simulink model "Sim_DDPG"  (R2025a)
settings: Solver=ode1  StartTime=0.0  StopTime=Tf  FixedStep=Ts_Sim  RelTol=1e-3
undefined symbols (not defined in the file): p_IC, phi_IC, phi_limit, pqr_Limit, psi_IC, psi_limit, q_IC, r_IC, theta_IC, theta_limit, Ts_Sim, u_IC, uvw_Limit, v_IC, w_IC, x_IC, xy_Limit, y_IC, z_IC, z_Limit
libraries: rllib x2
settings Model: Creator=nt488543  LastModifiedBy=nt488543

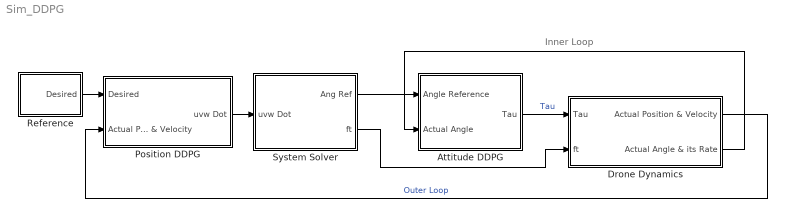
== system Sim_DDPG ==
  note: Inner Loop
  Attitude DDPG : Subsystem
  Drone Dynamics : Subsystem
  Position DDPG : Subsystem
  Reference : Subsystem
  System Solver : Subsystem
  wires:
  Reference/1(Desired) -> Position DDPG/1(Desired)
  Attitude DDPG/1(Tau) -> Drone Dynamics/1(Tau)  "Tau"
  Drone Dynamics/1(Actual Position & Velocity) -> Position DDPG/2(Actual Position & Velocity)  "Outer Loop"
  Drone Dynamics/2(Actual Angle & its Rate) -> Attitude DDPG/2(Actual Angle)
  Position DDPG/1(uvw Dot) -> System Solver/1(uvw Dot)
  System Solver/1(Ang Ref) -> Attitude DDPG/1(Angle Reference)
  System Solver/2(ft) -> Drone Dynamics/2(ft)

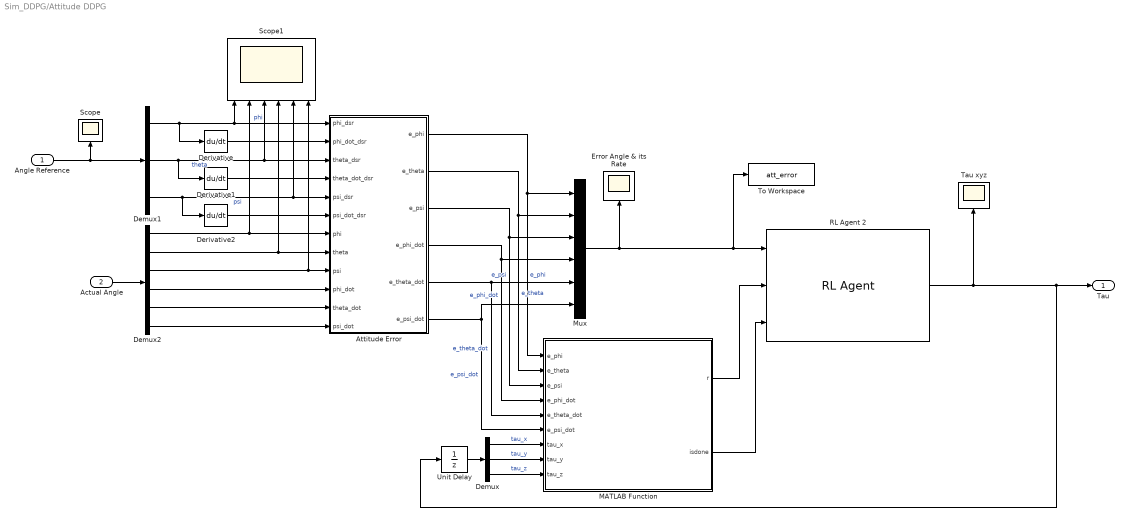
== system Sim_DDPG/Attitude DDPG ==
  Angle Reference : Inport
  Actual Angle : Inport  Port=2
  Attitude Error : MATLAB Function  TreatAsAtomicUnit=on
  Demux : Demux  Outputs=3
  Demux1 : Demux  Outputs=3
  Demux2 : Demux  Outputs=6
  Derivative : Derivative
  Derivative1 : Derivative
  Derivative2 : Derivative
  Error Angle & its Rate : Scope
      settings: ActiveDisplayYMinimum=-3.5181599273654109  ActiveDisplayYMaximum=2.1435969273697308  DataLoggingVariableName=ScopeData12
  MATLAB Function : MATLAB Function  TreatAsAtomicUnit=on
  Mux : Mux  Inputs=6
  RL Agent 2 : rllib/RL Agent  Agent=agent2  ExternalActionAsInput=off  ProvideLastAction=off  ProvideCumRwd=off  TreatAsDirectFeedthrough=on  UseStrictObservationDataTypes=off
  Scope : Scope
      settings: ActiveDisplayYMinimum=-0.07573  ActiveDisplayYMaximum=0.06612  DataLoggingVariableName=ScopeData5
  Scope1 : Scope  NumInputPorts=6
      settings: ActiveDisplayYMinimum=-0.31729729958403707  ActiveDisplayYMaximum=0.34620944603052173  DataLoggingVariableName=ScopeData6
  Tau xyz : Scope
      settings: ActiveDisplayYMinimum=-2.4987406879663467  ActiveDisplayYMaximum=2.4991613775491714  DataLoggingVariableName=ScopeData11
  To Workspace : ToWorkspace  VariableName=att_error  SampleTime=Ts_Sim
  Unit Delay : UnitDelay  SampleTime=Ts_Sim  HasFrameUpgradeWarning=on
  Tau : Outport
  wires:
  MATLAB Function/1(r) -> RL Agent 2/2
  Mux/1 -> To Workspace/1, RL Agent 2/1, Error Angle & its Rate/1
  Attitude Error/1(e_phi) -> Mux/1, MATLAB Function/1(e_phi)  "e_phi"
  Attitude Error/2(e_theta) -> Mux/2, MATLAB Function/2(e_theta)  "e_theta"
  Attitude Error/3(e_psi) -> Mux/3, MATLAB Function/3(e_psi)  "e_psi"
  Attitude Error/4(e_phi_dot) -> Mux/4, MATLAB Function/4(e_phi_dot)  "e_phi_dot"
  Attitude Error/5(e_theta_dot) -> MATLAB Function/5(e_theta_dot), Mux/5  "e_theta_dot"
  Attitude Error/6(e_psi_dot) -> MATLAB Function/6(e_psi_dot), Mux/6  "e_psi_dot"
  MATLAB Function/2(isdone) -> RL Agent 2/3
  Demux/1 -> MATLAB Function/7(tau_x)  "tau_x"
  Demux/2 -> MATLAB Function/8(tau_y)  "tau_y"
  Demux/3 -> MATLAB Function/9(tau_z)  "tau_z"
  RL Agent 2/1 -> Unit Delay/1, Tau/1, Tau xyz/1
  Demux2/1 -> Scope1/2, Attitude Error/7(phi)
  Demux2/2 -> Scope1/4, Attitude Error/8(theta)
  Demux2/3 -> Attitude Error/9(psi), Scope1/6
  Demux2/4 -> Attitude Error/10(phi_dot)
  Demux2/5 -> Attitude Error/11(theta_dot)
  Demux2/6 -> Attitude Error/12(psi_dot)
  Actual Angle/1 -> Demux2/1
  Unit Delay/1 -> Demux/1
  Demux1/1 -> Derivative/1, Attitude Error/1(phi_dsr), Scope1/1  "phi"
  Demux1/3 -> Derivative2/1, Attitude Error/5(psi_dsr), Scope1/5  "psi"
  Demux1/2 -> Derivative1/1, Attitude Error/3(theta_dsr), Scope1/3  "theta"
  Angle Reference/1 -> Demux1/1, Scope/1
  Derivative/1 -> Attitude Error/2(phi_dot_dsr)
  Derivative1/1 -> Attitude Error/4(theta_dot_dsr)
  Derivative2/1 -> Attitude Error/6(psi_dot_dsr)

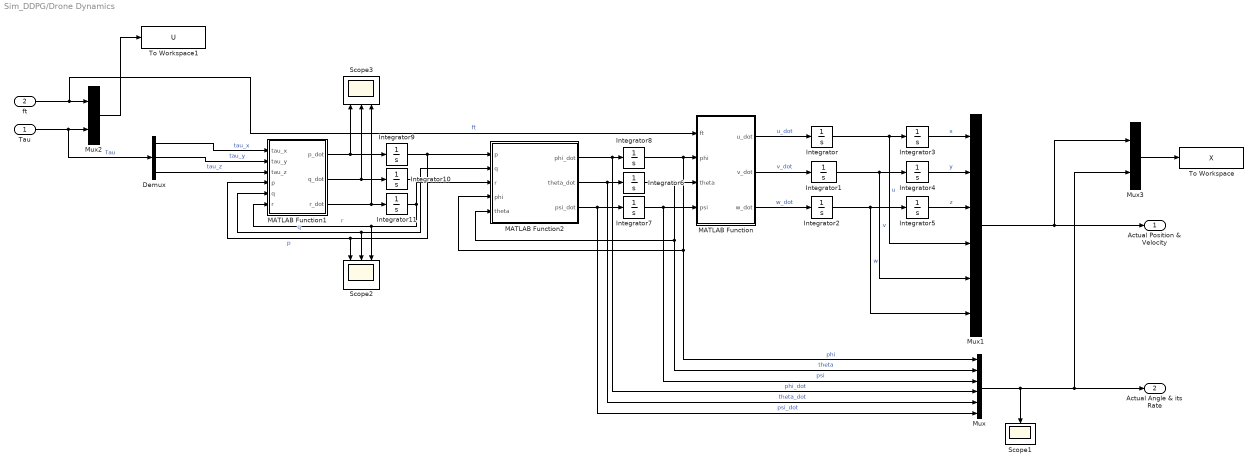
== system Sim_DDPG/Drone Dynamics ==
  Tau : Inport
  ft : Inport  Port=2
  Demux : Demux  Outputs=3
  Integrator : Integrator  InitialCondition=u_IC  UpperSaturationLimit=uvw_Limit  LowerSaturationLimit=-uvw_Limit
  Integrator1 : Integrator  InitialCondition=v_IC  UpperSaturationLimit=uvw_Limit  LowerSaturationLimit=-uvw_Limit
  Integrator10 : Integrator  InitialCondition=q_IC  UpperSaturationLimit=pqr_Limit  LowerSaturationLimit=-pqr_Limit
  Integrator11 : Integrator  InitialCondition=r_IC  UpperSaturationLimit=pqr_Limit  LowerSaturationLimit=-pqr_Limit
  Integrator2 : Integrator  InitialCondition=w_IC  UpperSaturationLimit=uvw_Limit  LowerSaturationLimit=-uvw_Limit
  Integrator3 : Integrator  InitialCondition=x_IC  UpperSaturationLimit=xy_Limit  LowerSaturationLimit=-xy_Limit
  Integrator4 : Integrator  InitialCondition=y_IC  UpperSaturationLimit=xy_Limit  LowerSaturationLimit=-xy_Limit
  Integrator5 : Integrator  InitialCondition=z_IC  UpperSaturationLimit=z_Limit  LowerSaturationLimit=-z_Limit
  Integrator6 : Integrator  InitialCondition=theta_IC  UpperSaturationLimit=theta_limit  LowerSaturationLimit=-theta_limit  WrappedStateUpperValue=pi/2  WrappedStateLowerValue=-pi/2
  Integrator7 : Integrator  InitialCondition=psi_IC  UpperSaturationLimit=psi_limit  LowerSaturationLimit=-psi_limit
  Integrator8 : Integrator  InitialCondition=phi_IC  UpperSaturationLimit=phi_limit  LowerSaturationLimit=-phi_limit
  Integrator9 : Integrator  InitialCondition=p_IC  UpperSaturationLimit=pqr_Limit  LowerSaturationLimit=-pqr_Limit
  MATLAB Function : MATLAB Function  TreatAsAtomicUnit=on
  MATLAB Function1 : MATLAB Function  TreatAsAtomicUnit=on
  MATLAB Function2 : MATLAB Function  TreatAsAtomicUnit=on
  Mux : Mux  Inputs=6
  Mux1 : Mux  Inputs=6
  Mux2 : Mux  Inputs=2
  Mux3 : Mux  Inputs=2
  Scope1 : Scope
      settings: ActiveDisplayYMinimum=-0.79782557910284335  ActiveDisplayYMaximum=0.70695961840012789  DataLoggingVariableName=ScopeData2
  Scope2 : Scope  NumInputPorts=3
      settings: ActiveDisplayYMinimum=-0.95183  ActiveDisplayYMaximum=0.89979  DataLoggingVariableName=ScopeData3
  Scope3 : Scope  NumInputPorts=3
      settings: ActiveDisplayYMinimum=-1  ActiveDisplayYMaximum=1  DataLoggingVariableName=ScopeData4
  To Workspace : ToWorkspace  VariableName=X  SampleTime=Ts_Sim
  To Workspace1 : ToWorkspace  VariableName=U  SampleTime=Ts_Sim
  Actual Position & Velocity : Outport
  Actual Angle & its Rate : Outport  Port=2
  wires:
  Integrator4/1 -> Mux1/2  "y"
  MATLAB Function1/3(r_dot) -> Scope3/3, Integrator11/1
  MATLAB Function1/1(p_dot) -> Scope3/1, Integrator9/1
  Integrator3/1 -> Mux1/1  "x"
  Integrator5/1 -> Mux1/3  "z"
  Integrator1/1 -> Mux1/5, Integrator4/1  "v"
  Demux/2 -> MATLAB Function1/2(tau_y)  "tau_y"
  Integrator9/1 -> MATLAB Function1/4(p), Scope2/1, MATLAB Function2/1(p)  "p"
  Integrator11/1 -> MATLAB Function1/6(r), Scope2/3, MATLAB Function2/3(r)  "r"
  Integrator2/1 -> Mux1/6, Integrator5/1  "w"
  Integrator/1 -> Mux1/4, Integrator3/1  "u"
  Integrator7/1 -> Mux/3, MATLAB Function/4(psi)  "psi"
  Integrator8/1 -> Mux/1, MATLAB Function2/4(phi), MATLAB Function/2(phi)  "phi"
  Integrator6/1 -> MATLAB Function/3(theta), Mux/2, MATLAB Function2/5(theta)  "theta"
  Integrator10/1 -> MATLAB Function2/2(q), MATLAB Function1/5(q), Scope2/2  "q"
  Demux/3 -> MATLAB Function1/3(tau_z)  "tau_z"
  MATLAB Function/3(w_dot) -> Integrator2/1  "w_dot"
  MATLAB Function/1(u_dot) -> Integrator/1  "u_dot"
  MATLAB Function/2(v_dot) -> Integrator1/1  "v_dot"
  MATLAB Function1/2(q_dot) -> Scope3/2, Integrator10/1
  Demux/1 -> MATLAB Function1/1(tau_x)  "tau_x"
  MATLAB Function2/1(phi_dot) -> Mux/4, Integrator8/1  "phi_dot"
  MATLAB Function2/2(theta_dot) -> Mux/5, Integrator6/1  "theta_dot"
  MATLAB Function2/3(psi_dot) -> Mux/6, Integrator7/1  "psi_dot"
  Mux/1 -> Mux3/2, Actual Angle & its Rate/1, Scope1/1
  Mux1/1 -> Mux3/1, Actual Position & Velocity/1
  Mux2/1 -> To Workspace1/1
  ft/1 -> MATLAB Function/1(ft), Mux2/1  "ft"
  Tau/1 -> Demux/1, Mux2/2  "Tau"
  Mux3/1 -> To Workspace/1

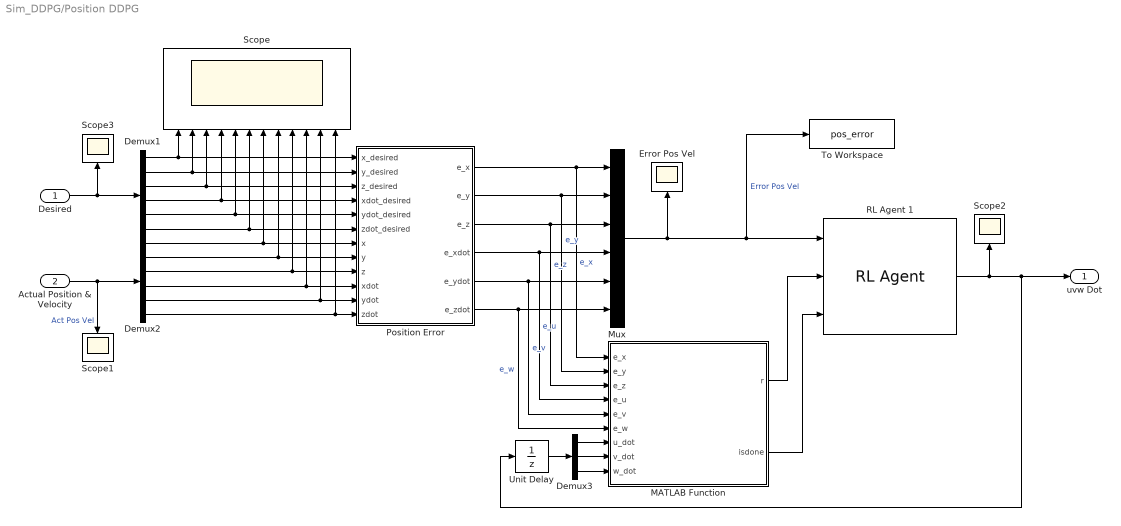
== system Sim_DDPG/Position DDPG ==
  Desired : Inport
  Actual Position & Velocity : Inport  Port=2
  Demux1 : Demux  Outputs=6
  Demux2 : Demux  Outputs=6
  Demux3 : Demux  Outputs=3
  Error Pos Vel : Scope
      settings: ActiveDisplayYMinimum=-1.3710264936743408  ActiveDisplayYMaximum=0.56946492466600562  DataLoggingVariableName=Error
  MATLAB Function : MATLAB Function  TreatAsAtomicUnit=on
  Mux : Mux  Inputs=6
  Position Error : MATLAB Function  TreatAsAtomicUnit=on
  RL Agent 1 : rllib/RL Agent  Agent=agent  ExternalActionAsInput=off  ProvideLastAction=off  ProvideCumRwd=off  TreatAsDirectFeedthrough=on  UseStrictObservationDataTypes=off
  Scope : Scope  NumInputPorts=12
      settings: ActiveDisplayYMinimum=-60.026881939696665  ActiveDisplayYMaximum=21.551746724254532  DataLoggingVariableName=Difference  DataLoggingSaveFormat=Structure
  Scope1 : Scope
      settings: ActiveDisplayYMinimum=-1313.1939544508978  ActiveDisplayYMaximum=197.10705078812913  DataLoggingVariableName=Actual
  Scope2 : Scope
      settings: ActiveDisplayYMinimum=-2.3417  ActiveDisplayYMaximum=1.0752  DataLoggingVariableName=ScopeData4
  Scope3 : Scope
      settings: ActiveDisplayYMinimum=-34.036737735877395  ActiveDisplayYMaximum=6.4906396228965306  DataLoggingVariableName=Ref
  To Workspace : ToWorkspace  VariableName=pos_error  SampleTime=Ts_Sim
  Unit Delay : UnitDelay  SampleTime=Ts_Sim  HasFrameUpgradeWarning=on
  uvw Dot : Outport
  wires:
  MATLAB Function/1(r) -> RL Agent 1/2
  Mux/1 -> To Workspace/1, RL Agent 1/1, Error Pos Vel/1  "Error Pos Vel"
  RL Agent 1/1 -> uvw Dot/1, Unit Delay/1, Scope2/1
  Position Error/1(e_x) -> MATLAB Function/1(e_x), Mux/1  "e_x"
  Position Error/2(e_y) -> MATLAB Function/2(e_y), Mux/2  "e_y"
  Position Error/3(e_z) -> Mux/3, MATLAB Function/3(e_z)  "e_z"
  Position Error/4(e_xdot) -> MATLAB Function/4(e_u), Mux/4  "e_u"
  Position Error/5(e_ydot) -> MATLAB Function/5(e_v), Mux/5  "e_v"
  Position Error/6(e_zdot) -> MATLAB Function/6(e_w), Mux/6  "e_w"
  MATLAB Function/2(isdone) -> RL Agent 1/3
  Demux1/1 -> Position Error/1(x_desired), Scope/1
  Demux1/2 -> Position Error/2(y_desired), Scope/2
  Demux1/3 -> Position Error/3(z_desired), Scope/3
  Demux1/4 -> Position Error/4(xdot_desired), Scope/4
  Demux1/5 -> Position Error/5(ydot_desired), Scope/5
  Demux1/6 -> Position Error/6(zdot_desired), Scope/6
  Desired/1 -> Scope3/1, Demux1/1
  Demux2/1 -> Position Error/7(x), Scope/7
  Demux2/2 -> Position Error/8(y), Scope/8
  Demux2/3 -> Position Error/9(z), Scope/9
  Demux2/4 -> Position Error/10(xdot), Scope/10
  Demux2/5 -> Position Error/11(ydot), Scope/11
  Demux2/6 -> Scope/12, Position Error/12(zdot)
  Actual Position & Velocity/1 -> Demux2/1, Scope1/1  "Act Pos Vel"
  Demux3/1 -> MATLAB Function/7(u_dot)
  Demux3/2 -> MATLAB Function/8(v_dot)
  Demux3/3 -> MATLAB Function/9(w_dot)
  Unit Delay/1 -> Demux3/1

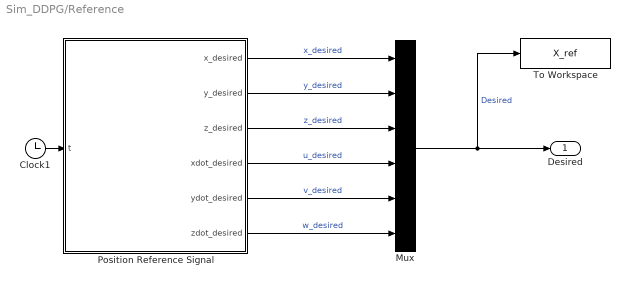
== system Sim_DDPG/Reference ==
  Clock1 : Clock
  Mux : Mux  Inputs=6
  Position Reference Signal : MATLAB Function  TreatAsAtomicUnit=on
  To Workspace : ToWorkspace  VariableName=X_ref  SampleTime=Ts_Sim
  Desired : Outport
  wires:
  Position Reference Signal/2(y_desired) -> Mux/2  "y_desired"
  Position Reference Signal/4(xdot_desired) -> Mux/4  "u_desired"
  Position Reference Signal/6(zdot_desired) -> Mux/6  "w_desired"
  Clock1/1 -> Position Reference Signal/1(t)
  Position Reference Signal/3(z_desired) -> Mux/3  "z_desired"
  Position Reference Signal/1(x_desired) -> Mux/1  "x_desired"
  Position Reference Signal/5(ydot_desired) -> Mux/5  "v_desired"
  Mux/1 -> To Workspace/1, Desired/1  "Desired"

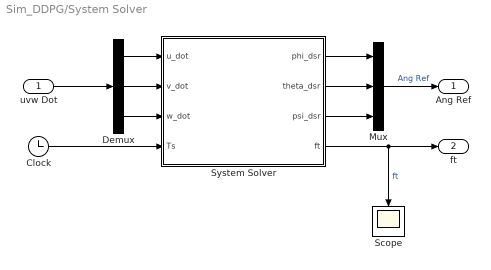
== system Sim_DDPG/System Solver ==
  uvw Dot : Inport
  Clock : Clock
  Demux : Demux  Outputs=3
  Mux : Mux  Inputs=3
  Scope : Scope
      settings: ActiveDisplayYMinimum=5.5477079741609581  ActiveDisplayYMaximum=13.965080226414941
  System Solver : MATLAB Function  TreatAsAtomicUnit=on
  Ang Ref : Outport
  ft : Outport  Port=2
  wires:
  System Solver/2(theta_dsr) -> Mux/2
  Demux/1 -> System Solver/1(u_dot)
  System Solver/3(psi_dsr) -> Mux/3
  Demux/2 -> System Solver/2(v_dot)
  System Solver/1(phi_dsr) -> Mux/1
  Demux/3 -> System Solver/3(w_dot)
  System Solver/4(ft) -> ft/1, Scope/1  "ft"
  Clock/1 -> System Solver/4(Ts)
  Mux/1 -> Ang Ref/1  "Ang Ref"
  uvw Dot/1 -> Demux/1

== matlab function Sim_DDPG/Position DDPG/Position Error ==
  data: x_desired input; y_desired input; z_desired input; xdot_desired input; ydot_desired input; zdot_desired input; x input; y input; z input; e_x output; e_y output; e_z output; xdot input; ydot input; zdot input; e_xdot output; e_ydot output; e_zdot output
function [e_x, e_y, e_z, e_xdot, e_ydot, e_zdot] = ...
      calculate_errors(x_desired, y_desired, z_desired, ...
      xdot_desired, ydot_desired, zdot_desired, ...
      x,y,z, xdot,ydot,zdot)

    e_x    = x_desired - x;
    e_y    = y_desired - y;
    e_z    = z_desired - z;
    e_xdot = xdot_desired - xdot;
    e_ydot = ydot_desired - ydot;
    e_zdot = zdot_desired - zdot;
    
end

% formal is Actual - Reference

== matlab function Sim_DDPG/Position DDPG/MATLAB Function ==
  data: e_x input; r output; e_y input; e_z input; e_u input; e_v input; e_w input; u_dot input; v_dot input; w_dot input; isdone output
function [r,isdone] = calculate_reward(e_x, e_y, e_z, e_u, e_v, e_w, u_dot, v_dot, w_dot)

    r = -    1*( abs(e_x)   + abs(e_y)   + abs(e_z) ) ...
        -  0.1*( abs(e_u)   + abs(e_v)   + abs(e_w) ) ...
        - 0.01*( abs(u_dot) + abs(v_dot) + abs(w_dot) );
    
   isdone = 0;
   
end

== matlab function Sim_DDPG/Attitude DDPG/MATLAB Function ==
  data: e_phi input; r output; e_theta input; e_psi input; e_phi_dot input; e_theta_dot input; e_psi_dot input; tau_x input; tau_y input; tau_z input; isdone output
function [r,isdone] = calculate_reward(e_phi, e_theta, e_psi, e_phi_dot, e_theta_dot, e_psi_dot, tau_x, tau_y, tau_z )

    Error_Angle      =    2*( abs(e_phi)     +  abs(e_theta)     + abs(e_psi) );
    Error_Angle_Rate =  0.1*( abs(e_phi_dot) +  abs(e_theta_dot) + abs(e_psi_dot) );
    Action           = 0.01*( abs(tau_x)     +  abs(tau_y)       + abs(tau_z) );

    r = - Error_Angle - Error_Angle_Rate - Action;

    isdone = (abs(e_phi) > 100) || (abs(e_theta) > 100) || (abs(e_psi) > 100);
end

== matlab function Sim_DDPG/Drone Dynamics/MATLAB Function1 ==
  data: tau_x input; p_dot output; tau_y input; tau_z input; p input; q_dot output; r_dot output; q input; r input
function [p_dot, q_dot, r_dot] = fcn(tau_x,tau_y,tau_z,p,q,r)

Ix = 0.3; Iy = 0.4; Iz = 0.5; 

p_dot = ((Iy-Iz)*q*r/Ix)  + tau_x/Ix;
q_dot = ((Iz-Ix)*p*r/Iy)  + tau_y/Iy;
r_dot = ((Ix-Iy)*p*q/Iz)  + tau_z/Iz;


end

== matlab function Sim_DDPG/Drone Dynamics/MATLAB Function ==
  data: ft input; u_dot output; phi input; theta input; psi input; v_dot output; w_dot output
function [u_dot, v_dot, w_dot] = fcn(ft,phi,theta,psi)

m = 1; g = 9.81;

u_dot = -(ft/m)*( sin(phi)*sin(psi) + cos(phi)*cos(psi)*sin(theta) ); 
v_dot = -(ft/m)*( cos(phi)*sin(psi)*sin(theta) - cos(psi)*sin(phi));
w_dot = g-(ft/m)*( cos(phi)*cos(theta) );

end

== matlab function Sim_DDPG/Drone Dynamics/MATLAB Function2 ==
  data: p input; q input; r input; phi_dot output; phi input; theta input; theta_dot output; psi_dot output
function [phi_dot, theta_dot, psi_dot] = fcn(p,q,r, phi,theta)

    phi_dot   = p + (q*sin(phi)*tan(theta)) + (r*cos(phi)*tan(theta));
    theta_dot = (q*cos(phi)) - (r*sin(phi));
    psi_dot   = (q*sin(phi)/cos(theta)) + (r*cos(phi)/cos(theta));

end



    % if theta == deg2rad(90) || theta == deg2rad(-90)
    %    theta = sign(theta)*deg2rad(89.9); 
    % end

% 89.9 value is fixed. 
% if change to 89.99, phi_dot and psi_dot value will explode.

== matlab function Sim_DDPG/Reference/Position Reference Signal ==
  data: t input; x_desired output; y_desired output; z_desired output; xdot_desired output; ydot_desired output; zdot_desired output
function [x_desired, y_desired, z_desired, xdot_desired, ydot_desired, zdot_desired] = trajectory_generator(t)

    x_desired    = 9.81 * (1-exp(-0.01*t)) * cos(0.2*t);
    xdot_desired = 9.81 * ( (0.01*exp(-0.01*t)*cos(0.2*t)) - (0.2*(1-exp(-0.01*t))*sin(0.2*t)) );

    y_desired    = 9.81 * (1-exp(-0.01*t)) * sin(0.2*t);
    ydot_desired = 9.81 * ( (0.01*exp(-0.01*t)*sin(0.2*t)) + (0.2*(1-exp(-0.01*t))*cos(0.2*t)) );

    z_desired    = -1*t;
    zdot_desired = -1;

end


% ref = @(t) [(1-exp(-0.01*t))*9.81*cos(0.2*t);
%             (1-exp(-0.01*t))*9.81*sin(0.2*t);
%             -.1*t];


 % x_desired    = 9.81 * (1-exp(-0.01*t)) * cos(0.2*t);
 %    xdot_desired = 9.81 * ( (0.01*exp(-0.01*t)*cos(0.2*t)) - (0.2*(1-exp(-0.01*t))*sin(0.2*t)) );
 % 
 %    y_desired    = 9.81 * (1-exp(-0.01*t)) * sin(0.2*t);
 %    ydot_desired = 9.81 * ( (0.01*exp(-0.01*t)*sin(0.2*t)) + (0.2*(1-exp(-0.01*t))*cos(0.2*t)) );
 % 
 %    z_desired    = -0.1*t;
 %    zdot_desired = -0.1;

== matlab function Sim_DDPG/System Solver/System Solver ==
  data: phi_dsr output; theta_dsr output; psi_dsr output; ft output; u_dot input; v_dot input; w_dot input; Ts input
function [phi_dsr, theta_dsr,psi_dsr, ft ] = system_solver(u_dot, v_dot, w_dot, Ts)

    m = 1; g = 9.81; 

    ft = m * sqrt( u_dot^2 + v_dot^2 + (w_dot-g)^2 );
    
    phi_dsr = asin( (v_dot*m) / ft );
    theta_dsr = asin( (-u_dot*m) / (ft*cos(phi_dsr)) );
    psi_dsr = 0;

    % Smoothing Factor ( Use exponential decay, just to start from zero )
    phi_dsr = phi_dsr * (1-exp(-Ts));
    theta_dsr = theta_dsr * (1-exp(-Ts));
    psi_dsr = psi_dsr * (1-exp(-Ts));

    % Saturation
    if phi_dsr > pi/10
        phi_dsr = pi/10;
    elseif phi_dsr < -pi/10
        phi_dsr = -pi/10;
    end

    if theta_dsr > pi/10
        theta_dsr = pi/10;
    elseif theta_dsr < -pi/10
        theta_dsr = -pi/10;
    end

end

== matlab function Sim_DDPG/Attitude DDPG/Attitude Error ==
  data: phi_dsr input; phi_dot_dsr input; theta_dsr input; theta_dot_dsr input; psi_dsr input; psi_dot_dsr input; phi input; theta input; psi input; e_phi output; e_theta output; e_psi output; phi_dot input; theta_dot input; psi_dot input; e_phi_dot output; e_theta_dot output; e_psi_dot output
function [ e_phi, e_theta, e_psi, e_phi_dot, e_theta_dot, e_psi_dot ] = calculate_errors(phi_dsr, phi_dot_dsr, theta_dsr, theta_dot_dsr, psi_dsr, psi_dot_dsr, phi, theta, psi, phi_dot, theta_dot, psi_dot)
   
    e_phi = phi_dsr - phi;
    e_theta = theta_dsr - theta;
    e_psi = psi_dsr - psi;

    e_phi_dot = phi_dot_dsr - phi_dot;
    e_theta_dot = theta_dot_dsr - theta_dot;
    e_psi_dot = psi_dot_dsr - psi_dot;

end
